simulink model "water_hammer"  (R2020a)
settings: Solver=ode15s  StartTime=0.0  StopTime=30  RelTol=1e-3  AbsTol=1e-3
undefined symbols (not defined in the file or in its folder): mdot0, p0
libraries: fl_lib x11, nesl_utility x5, SimscapeFluids_lib x1, simulink x1
settings Model: Creator=Afraz  LastModifiedBy=Afraz
settings SolverCC: AutoScaleAbsTol=off
settings DebuggingCC: SymbolicDimsDataTypeCodeGenerationDiagnostic=none
settings SFSimCC: CustomCodeUndefinedFunction=UseInterfaceOnly
settings SimscapeCC: SimscapeLogType=all  SimscapeLogSimulationStatistics=on  SimscapeLogDataHistory=10000

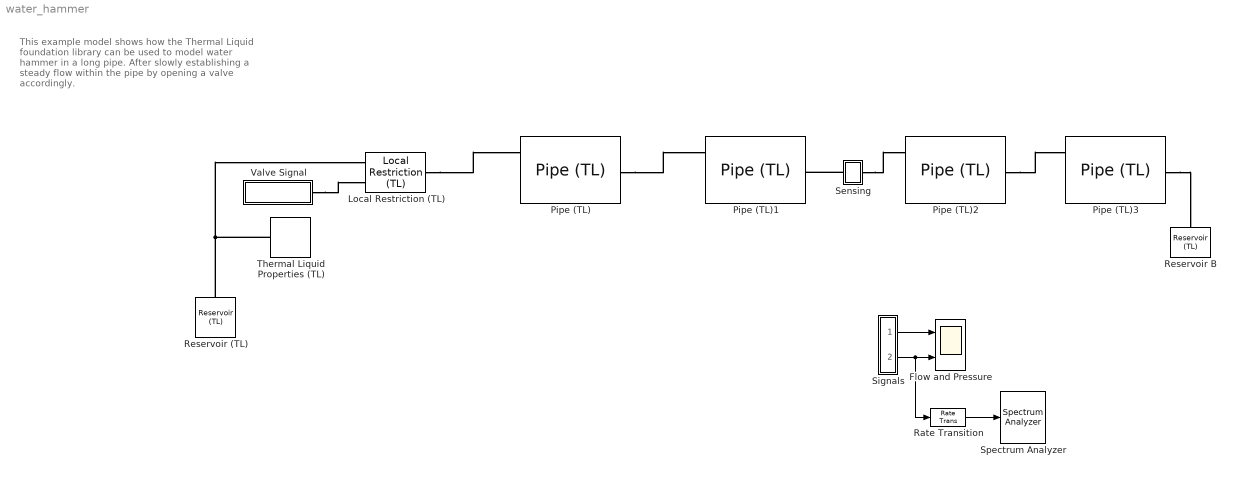
== system water_hammer ==
  note: This example model shows how the Thermal Liquid foundation library can be used to model water hammer in a long pipe. After slowly establishing a steady flow within the pipe by opening a valve accordingly.
  Flow and Pressure : Scope  NumInputPorts=2
  Local Restriction (TL) : fl_lib/Thermal Liquid/Elements/Local Restriction (TL)  restriction_type=foundation.enum.restriction_type.variable  restriction_area=0.001 m^2  min_area=1e-10 m^2  max_area=0.005 m^2  area=0.01 m^2  Cd=0.64  pressure_recovery=simscape.enum.onoff.on  Re_c=12
      settings: SourceProductBaseCode=SS  InternalSimscapePortConfiguration="{\"Bottom\":[],\"Left\":[{\"id\":\"A\",\"label\":\"A\",\"type\":\"foundation.thermal_liquid.thermal_liquid\"},{\"id\":\"area_in\",\"label\":\"AR\",\"type\":\"input\"}],\"Right\":[{\"id\":\"B\",\"label\":\"B\",\"type\":\"foundation.thermal_liquid.thermal_liquid\"}],\"Top\":[]}"
  Pipe (TL){,1..3} (4 alike) : fl_lib/Thermal Liquid/Elements/Pipe (TL)  length=30/4 m  area=0.01 m^2  Dh=0.1128 m  length_add=1 m  roughness=15e-6 m  Re_lam=2000  Re_tur=4000  shape_factor=64  Nu_lam=3.66  dynamic_compressibility=simscape.enum.onoff.on  inertia=simscape.enum.onoff.off  p0=0.101325 MPa  T0=293.15 K  mdot0=0 kg/s
      settings: SourceProductBaseCode=SS
  Rate Transition : RateTransition  OutPortSampleTime=.0016
  Reservoir (TL) : fl_lib/Thermal Liquid/Elements/Reservoir (TL)  pressure_spec=foundation.enum.pressure_spec.specified  reservoir_pressure=6 bar  reservoir_temperature=293.15 K  area=0.01 m^2
      settings: SourceProductBaseCode=SS
  Reservoir B : fl_lib/Thermal Liquid/Elements/Reservoir (TL)  pressure_spec=foundation.enum.pressure_spec.specified  reservoir_pressure=5 bar  reservoir_temperature=293.15 K  area=.010 m^2
      settings: SourceProductBaseCode=MT,SS
  Sensing : Subsystem
      mask Display: disp('S')
  Signals : Subsystem
      mask Display: disp('S')
  Spectrum Analyzer : SpectrumAnalyzer
  Thermal Liquid Properties (TL) : SimscapeFluids_lib/Thermal Liquid/Utilities/Thermal Liquid Properties (TL)  fluid_list=fluids.thermal_liquid.utilities.enum.thermal_liquid_fluid_list.water  concentration_param_EG=fluids.thermal_liquid.utilities.enum.thermal_liquid_concentration.volume_fraction  concentration_param_PG=fluids.thermal_liquid.utilities.enum.thermal_liquid_concentration.volume_fraction  c_mass_SW=3.5e-3  c_mass_EG=0.1  c_mass_PG=0.1  c_mass_GL=0.1  c_vol_EG=0.1  c_vol_PG=0.1  beta_const_EG=2.1791 GPa  beta_const_PG=2.1791 GPa  beta_const_GL=2.1791 GPa  p_min_EG=0.01 MPa  p_min_PG=0.01 MPa  p_min_GL=0.01 MPa  p_max_EG=50 MPa  p_max_PG=50 MPa  p_max_GL=50 MPa  p_atm=0.101325 MPa
      settings: SourceProductBaseCode=SH
  Valve Signal : Subsystem  mask(Configure Valve Signal){valve_fastslow=Fast}
      mask prompts: valve_fastslow "Valve Closing Speed"
      mask help:
      | Select "Slow" to close the valve in 1 second.
      | Select "Fast" to close the valve in 10 ms.
      mask init:
      | if strcmp(get_param(gcb,'valve_fastslow'),'Slow')
      |     set_param([gcb '/S-PS Close Valve'],'InputFilterTimeConstant','1');
      | elseif strcmp(get_param(gcb,'valve_fastslow'),'Fast')
      |     set_param([gcb '/S-PS Close Valve'],'InputFilterTimeConstant','0.01');
      | end
      | set_param(gcb,'MaskDisplay',['disp(''' get_param(gcb,'valve_fastslow') ''');']);
      mask TypeOptions valve_fastslow: Slow | Fast
      mask Display: disp('Fast');
  wires:
  Rate Transition/1 -> Spectrum Analyzer/1
  Signals/1(mdot) -> Flow and Pressure/1
  Signals/2(p) -> Rate Transition/1, Flow and Pressure/2
  connections:
  Reservoir (TL)/LConn1 -- Thermal Liquid Properties (TL)/RConn1 -- Local Restriction (TL)/LConn1
  Valve Signal/RConn1 -- Local Restriction (TL)/LConn2
  Local Restriction (TL)/RConn1 -- Pipe (TL)/LConn1
  Pipe (TL)/RConn1 -- Pipe (TL)1/LConn1
  Sensing/LConn1 -- Pipe (TL)1/RConn1
  Sensing/RConn1 -- Pipe (TL)2/LConn1
  Pipe (TL)2/RConn1 -- Pipe (TL)3/LConn1
  Pipe (TL)3/RConn1 -- Reservoir B/LConn1

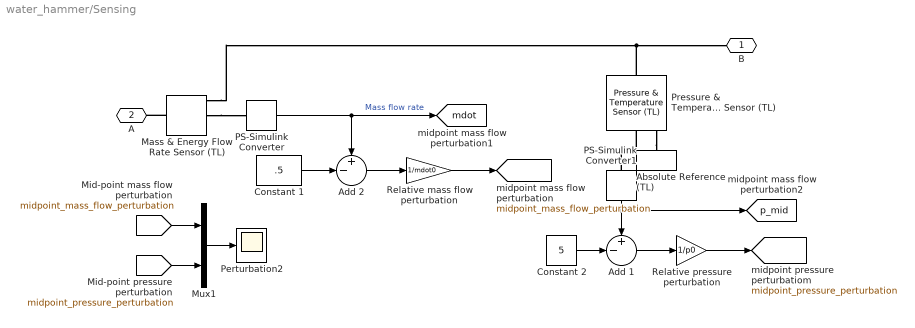
== system water_hammer/Sensing ==
  Absolute Reference (TL) : fl_lib/Thermal Liquid/Elements/Absolute Reference (TL)
      settings: SourceProductBaseCode=MT,SS
  Add 1 : Sum  Inputs=+-|
  Add 2 : Sum  Inputs=+-|
  Constant 1 : Constant  Value=.5
  Constant 2 : Constant  Value=5
  Mass & Energy Flow Rate Sensor (TL) : fl_lib/Thermal Liquid/Sensors/Mass & Energy Flow Rate Sensor (TL)
      settings: SourceProductBaseCode=MT,SS  InternalSimscapePortConfiguration="{\"Bottom\":[],\"Left\":[{\"id\":\"A\",\"label\":\"A\",\"type\":\"foundation.thermal_liquid.thermal_liquid\"}],\"Right\":[{\"id\":\"B\",\"label\":\"B\",\"type\":\"foundation.thermal_liquid.thermal_liquid\"},{\"id\":\"M\",\"label\":\"M\",\"type\":\"output\"},{\"id\":\"PHI\",\"label\":\"Phi\",\"type\":\"output\"}],\"Top\":[]}"
  Mux1 : Mux  Inputs=2
  PS-Simulink Converter : nesl_utility/PS-Simulink Converter  PhysicalDomain=network_engine_domain  SubClassName=ps_output  LeftPortType=input  RightPortType=output  PseudoPeriodic=off  Frequencies=[]  Unit=1  AffineConversion=off
      settings: SourceProductBaseCode=MT,SS
  PS-Simulink Converter1 : nesl_utility/PS-Simulink Converter  PhysicalDomain=network_engine_domain  SubClassName=ps_output  LeftPortType=input  RightPortType=output  PseudoPeriodic=off  Frequencies=[]  Unit=bar  AffineConversion=off
      settings: SourceProductBaseCode=MT,SS
  Perturbation2 : Scope
  Pressure & Temperature Sensor (TL) : fl_lib/Thermal Liquid/Sensors/Pressure & Temperature Sensor (TL)
      settings: SourceProductBaseCode=MT,SS  InternalSimscapePortConfiguration="{\"Bottom\":[],\"Left\":[{\"id\":\"A\",\"label\":\"A\",\"type\":\"foundation.thermal_liquid.thermal_liquid\"}],\"Right\":[{\"id\":\"B\",\"label\":\"B\",\"type\":\"foundation.thermal_liquid.thermal_liquid\"},{\"id\":\"P\",\"label\":\"P\",\"type\":\"output\"},{\"id\":\"T\",\"label\":\"T\",\"type\":\"output\"}],\"Top\":[]}"
  Relative mass flow perturbation : Gain  Gain=1/mdot0
  Relative pressure perturbation : Gain  Gain=1/p0
  B : PMIOPort  Side=Right
  A : PMIOPort  Port=2  Side=Left
  tag scope: mdot=global, midpoint_mass_flow_perturbation=global, midpoint_pressure_perturbation=global, p_mid=global
  wires:
  Constant 1/1 -> Add 2/2
  PS-Simulink Converter/1 -> [mdot], Add 2/1  "Mass flow rate"
  Add 2/1 -> Relative mass flow perturbation/1
  Relative mass flow perturbation/1 -> [midpoint_mass_flow_perturbation]
  Relative pressure perturbation/1 -> [midpoint_pressure_perturbation]
  Add 1/1 -> Relative pressure perturbation/1
  PS-Simulink Converter1/1 -> [p_mid], Add 1/1
  Constant 2/1 -> Add 1/2
  [midpoint_pressure_perturbation] -> Mux1/2
  [midpoint_mass_flow_perturbation] -> Mux1/1
  Mux1/1 -> Perturbation2/1
  connections:
  Mass & Energy Flow Rate Sensor (TL)/RConn1 -- Pressure & Temperature Sensor (TL)/LConn1 -- B/RConn1
  Mass & Energy Flow Rate Sensor (TL)/RConn2 -- PS-Simulink Converter/LConn1
  Mass & Energy Flow Rate Sensor (TL)/LConn1 -- A/RConn1
  Pressure & Temperature Sensor (TL)/RConn1 -- Absolute Reference (TL)/LConn1
  PS-Simulink Converter1/LConn1 -- Pressure & Temperature Sensor (TL)/RConn2

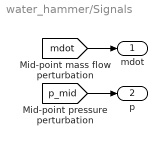
== system water_hammer/Signals ==
  mdot : Outport  VectorParamsAs1DForOutWhenUnconnected=off
  p : Outport  Port=2  VectorParamsAs1DForOutWhenUnconnected=off
  wires:
  [p_mid] -> p/1
  [mdot] -> mdot/1

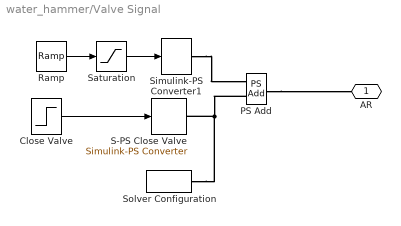
== system water_hammer/Valve Signal ==
  Close Valve : Step  Time=20  Before=2.55e-5  After=-2.55e-5  SampleTime=0
  PS Add : fl_lib/Physical Signals/Functions/PS Add
      settings: SourceProductBaseCode=MT,SS
  Ramp : simulink/Sources/Ramp  slope=2.55e-5/5  start=2  InitialOutput=-2.55e-5
  S-PS Close Valve : nesl_utility/Simulink-PS Converter  Tag=CustomStyle  PhysicalDomain=network_engine_domain  SubClassName=ps_input  LeftPortType=input  RightPortType=output  PseudoPeriodic=off  Frequencies=[]  NoiseDistribution=none  NoiseParameters=[]  Unit=m^2  AffineConversion=off  FilteringAndDerivatives=filter  SimscapeFilterOrder=1  InputFilterTimeConstant=0.01  UdotUserProvided=1
      settings: AttributesFormatString=Tau=%<InputFilterTimeConstant>(s)  SourceProductBaseCode=MT,SS
  Saturation : Saturate  UpperLimit=2.55e-5  LowerLimit=-2.55e-5  ZeroCross=off
  Simulink-PS Converter1 : nesl_utility/Simulink-PS Converter  PhysicalDomain=network_engine_domain  SubClassName=ps_input  LeftPortType=input  RightPortType=output  PseudoPeriodic=off  Frequencies=[]  NoiseDistribution=none  NoiseParameters=[]  Unit=m^2  AffineConversion=off  FilteringAndDerivatives=filter  SimscapeFilterOrder=1  InputFilterTimeConstant=1  UdotUserProvided=1
      settings: SourceProductBaseCode=MT,SS
  Solver Configuration : nesl_utility/Solver Configuration  PhysicalDomain=network_engine_domain  SubClassName=solver  LeftPortType=input  RightPortType=generic  Tones=[]  Harmonics=[]  SimulateNoise=off  Profile=off  UseLocalSampling=off  EnableSwitchedLinearOptims=on  FrequencyDomain=off  UseCCode=off  RelTol=0.001  AbsTol=1e-06  MinStep=1e-09  ToWorkspace=off  RevertToSquareIcSolve=off  NumHomotopyIterations=100  PhasorMode=off  PhasorModeNumHarmonics=1  DoDC=off  ResidualTolerance=1e-10  UseLocalSolver=off  LocalSolverChoice=NE_TRAPEZOIDAL_ADVANCER  LocalSolverSampleTime=0.001  DoFixedCost=off  MaxNonlinIter=3  MaxModeIter=2  LinearAlgebra=Sparse  EquationFormulation=NE_TIME_EF  DelaysMemoryBudget=1024  AutomaticFiltering=on  FilteringTimeConstant=0.001  PartitionStorageMethod=AS_NEEDED  PartitionMemoryBudget=1024  PartitionMethod=FAST
      settings: SourceProductBaseCode=MT,SS
  AR : PMIOPort  Side=Right
  wires:
  Close Valve/1 -> S-PS Close Valve/1
  Ramp/1 -> Saturation/1
  Saturation/1 -> Simulink-PS Converter1/1
  connections:
  PS Add/RConn1 -- AR/RConn1
  PS Add/LConn2 -- Solver Configuration/RConn1 -- S-PS Close Valve/RConn1
  Simulink-PS Converter1/RConn1 -- PS Add/LConn1
